simulink model "estimate_doppler_model"  (R2020a)
settings: Solver=VariableStepAuto  StartTime=0.0  StopTime=15  RelTol=1e-3
libraries: dspspect3 x1, dspsigops x1, dspsrcs4 x1
settings Model: Creator=juanj  LastModifiedBy=juanj

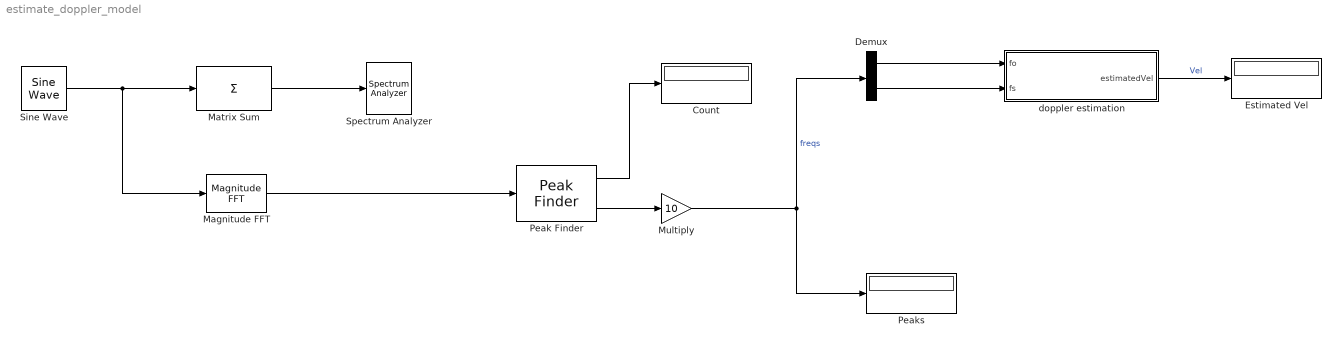
== system estimate_doppler_model ==
  Count : Display
  Demux : Demux  Outputs=2
  Estimated Vel : Display
  Magnitude FFT : dspspect3/Magnitude FFT  mag_or_magsq=Magnitude squared  FFTImplementation=Auto  fftLenInherit=off  fftsize=1000  WrapInput=on
      settings: SourceProductBaseCode=DS
  Matrix Sum : Sum  Inputs=+  CollapseMode=Specified dimension  CollapseDim=2
  Multiply : Gain  Gain=10  OutDataTypeStr=double  ParamDataTypeStr=Inherit: Same as input
  Peak Finder : dspsigops/Peak Finder  polarity=Maxima  outputIdx=on  outputVal=off  maxPeaks=1  NoiseDistinguish=off  thresh=0  roundingMode=Floor  overflowMode=off
      settings: SourceProductBaseCode=DS  allowOverrides=off
  Peaks : Display
      settings: Decimation=2
  Sine Wave : dspsrcs4/Sine Wave  Amplitude=1  Frequency=[1520 1600]  Phase=0  SampleMode=Discrete  OutComplex=Complex  CompMethod=Trigonometric fcn  TableSize=Speed  SampleTime=1/10000  SamplesPerFrame=2  ResetState=Restart at time zero  OutputFrames=off  dataType=double  wordLen=16  udDataType=sfix(16)  fracBitsMode=Best precision  numFracBits=15  OutDataTypeStr=double  LastOutDataTypeStr=double
  Spectrum Analyzer : SpectrumAnalyzer
  doppler estimation : MATLAB Function  TreatAsAtomicUnit=on
  wires:
  Sine Wave/1 -> Magnitude FFT/1, Matrix Sum/1
  Matrix Sum/1 -> Spectrum Analyzer/1
  Peak Finder/2 -> Multiply/1
  Magnitude FFT/1 -> Peak Finder/1
  Multiply/1 -> Demux/1, Peaks/1  "freqs"
  doppler estimation/1(estimatedVel) -> Estimated Vel/1  "Vel"
  Peak Finder/1 -> Count/1
  Demux/2 -> doppler estimation/2(fs)
  Demux/1 -> doppler estimation/1(fo)

== matlab function estimate_doppler_model/doppler estimation ==
  data: fo input; fs input; estimatedVel output
function estimatedVel = fcn(fo, fs)
%#codegen
c = 2.997e8; % Velocidad de la luz
estimatedVel = (c*fs)/fo - c; % Fórmula del efecto Doppler
